simulink model "W1P4"  (R2020b)
settings: Solver=VariableStepAuto  StartTime=0.0  StopTime=0.1  RelTol=1e-3
settings Model: Creator=saadh  LastModifiedBy=saadh

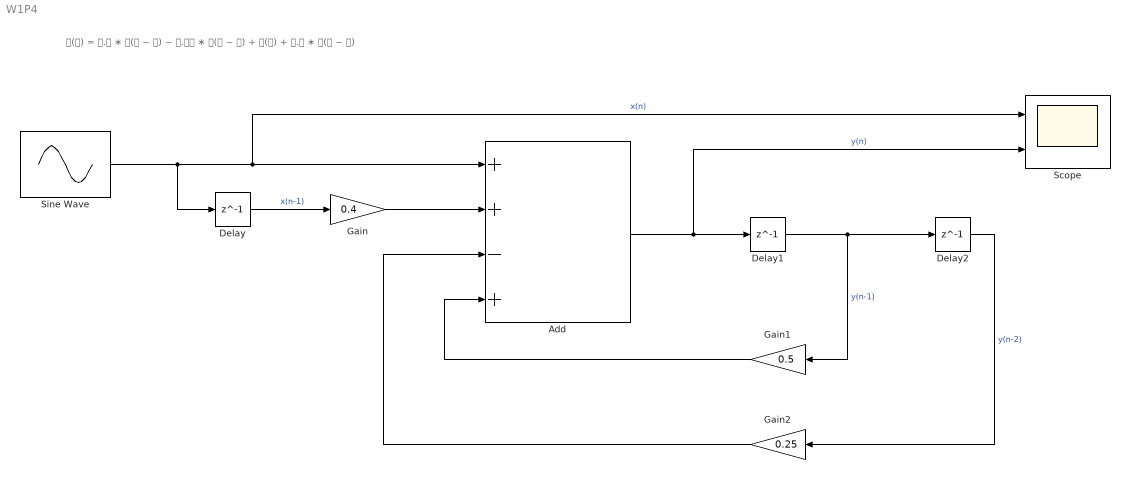
== system W1P4 ==
  note: 𝐲(𝐧) = 𝟎.𝟓 ∗ 𝐲(𝐧 − 𝟏) − 𝟎.𝟐𝟓 ∗ 𝐲(𝐧 − 𝟐) + 𝐱(𝐧) + 𝟎.𝟒 ∗ 𝐱(𝐧 − 𝟏)
  Add : Sum  Inputs=++-+
  Delay : Delay  DelayLength=1
  Delay1 : Delay  DelayLength=1
  Delay2 : Delay  DelayLength=1
  Gain : Gain  Gain=0.4
  Gain1 : Gain  Gain=0.5
  Gain2 : Gain  Gain=0.25
  Scope : Scope  NumInputPorts=2
  Sine Wave : Sin  Frequency=2*pi*100  SampleTime=0
  wires:
  Sine Wave/1 -> Delay/1, Scope/1, Add/1  "x(n)"
  Gain/1 -> Add/2
  Delay/1 -> Gain/1  "x(n-1)"
  Add/1 -> Scope/2, Delay1/1  "y(n)"
  Delay1/1 -> Gain1/1, Delay2/1  "y(n-1)"
  Gain1/1 -> Add/4
  Delay2/1 -> Gain2/1  "y(n-2)"
  Gain2/1 -> Add/3
